simulink model "SampleSimulinkModel"  (R2024a)
settings: Solver=FixedStepAuto  StartTime=0.0  StopTime=inf  RelTol=1e-3
settings Model: Creator=test-bed  LastModifiedBy=tagray
settings OptimizationCC: DefaultParameterBehavior=Inlined  EnhancedBackFolding=on  PassReuseOutputArgsAs=Individual arguments  ZeroExternalMemoryAtStartup=off  ZeroInternalMemoryAtStartup=off  OptimizeBlockOrder=speed  DifferentSizesBufferReuse=on  OptimizationCustomize=off  EfficientTunableParamExpr=on
settings DebuggingCC: ParameterTunabilityLossMsg=error
settings SFSimCC: MATLABDynamicMemAlloc=off
settings RTWCC: Description=Embedded Coder  SystemTargetFile=ert.tlc  TemplateMakefile=ert_default_tmf  CustomHeaderCode=cross_ipc.h  Toolchain=Microsoft Visual C++ 2022 v17.0 | nmake (64-bit Windows)  BuildConfiguration=Specify  TargetLang=C++
settings RTWCC: CustomSource=|
  | cross_ipc.c
  | sfun_connector.c
settings CodeAppCC: ForceParamTrailComments=on  IgnoreCustomStorageClasses=off  OperatorAnnotations=on  SimulinkDataObjDesc=on  SFDataObjDesc=on  InsertBlockDesc=on
settings ERTTargetCC: TargetLangStandard=C++11 (ISO)  GenerateSampleERTMain=on  CodeInterfacePackaging=C++ class  SupportContinuousTime=on  SupportNonInlinedSFcns=on  InlinedParameterPlacement=NonHierarchical  RootIOFormat=Structure reference  ERTCustomFileTemplate=example_file_process.tlc

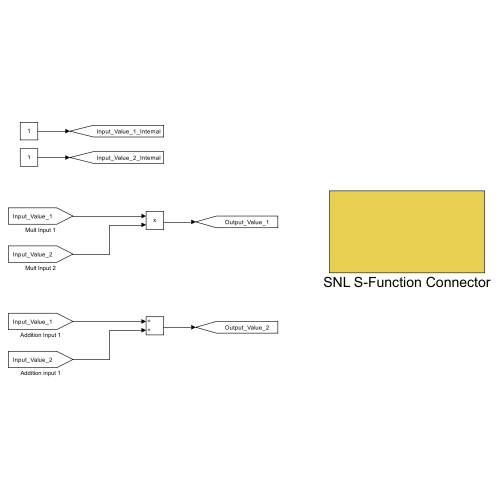
[thumbnail: Simulink's stored preview of the top-level diagram]
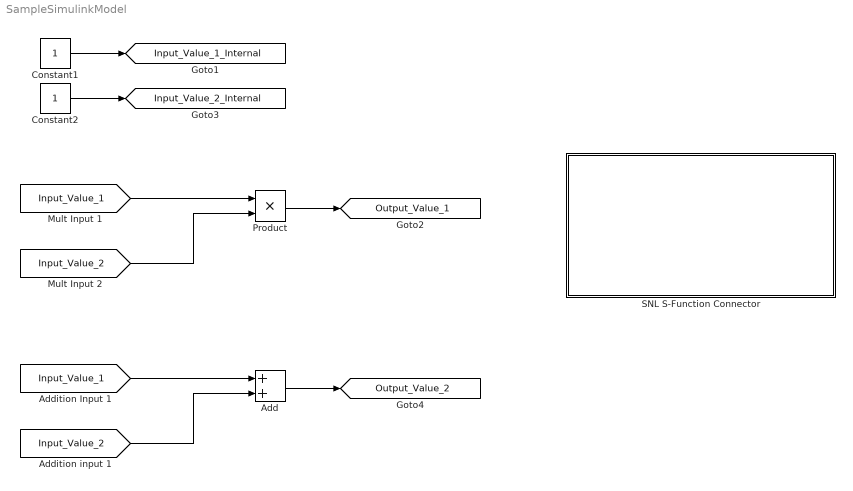
== system SampleSimulinkModel ==
  Add : Sum
  Constant1 : Constant
  Constant2 : Constant
  Product : Product
  SNL S-Function Connector : Subsystem
  tag scope: Input_Value_1_Internal=global, Input_Value_2_Internal=global, Output_Value_1=global, Output_Value_2=global
  wires:
  Constant1/1 -> [Input_Value_1_Internal]
  [Input_Value_1] -> Product/1
  [Input_Value_2] -> Product/2
  Product/1 -> [Output_Value_1]
  Constant2/1 -> [Input_Value_2_Internal]
  [Input_Value_2] -> Add/2
  Add/1 -> [Output_Value_2]
  [Input_Value_1] -> Add/1

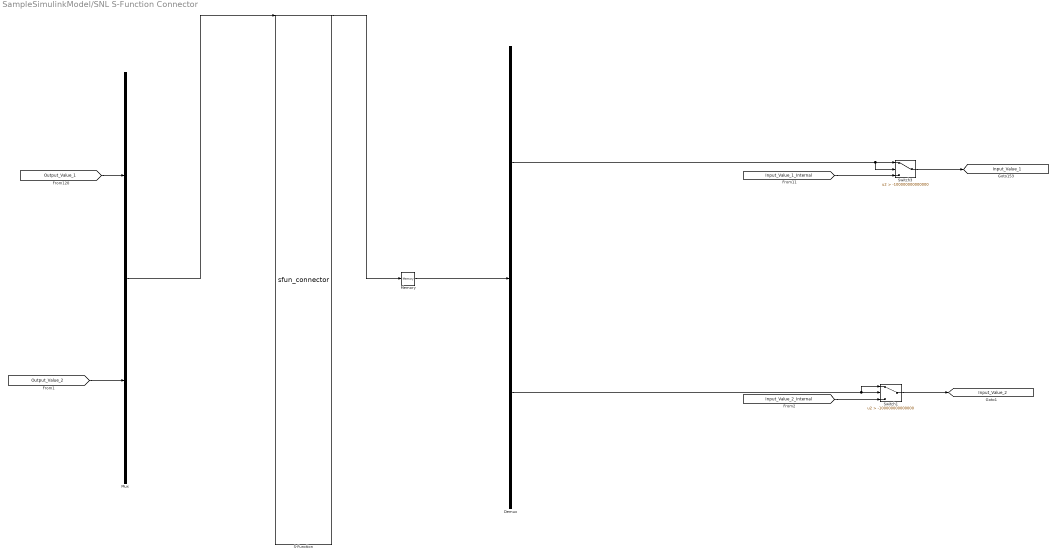
== system SampleSimulinkModel/SNL S-Function Connector ==
  Demux : Demux  Outputs=2
  Memory : Memory  InitialCondition=-100000000000000
  Mux : Mux  Inputs=2
  S-Function : S-Function  FunctionName=sfun_connector  Parameters='Output_Value_1;Output_Value_2','Input_Value_1;Input_Value_2'  SFunctionDeploymentMode=off  EnableBusSupport=off
  Switch1 : Switch  Criteria=u2 > Threshold  Threshold=-100000000000000  SaturateOnIntegerOverflow=off  InputSameDT=off
  Switch3 : Switch  Criteria=u2 > Threshold  Threshold=-100000000000000  SaturateOnIntegerOverflow=off  InputSameDT=off
  tag scope: Input_Value_1=global, Input_Value_2=global
  wires:
  [Output_Value_1] -> Mux/1
  Mux/1 -> S-Function/1
  Demux/1 -> Switch3/2, Switch3/1
  S-Function/1 -> Memory/1
  Switch3/1 -> [Input_Value_1]
  [Input_Value_1_Internal] -> Switch3/3
  Memory/1 -> Demux/1
  [Output_Value_2] -> Mux/2
  Switch1/1 -> [Input_Value_2]
  [Input_Value_2_Internal] -> Switch1/3
  Demux/2 -> Switch1/1, Switch1/2
